simulink model "q1"  (R2020b)
settings: Solver=VariableStepAuto  StartTime=0.0  StopTime=10.0  RelTol=1e-3
settings Model: Creator=MY lenovo  LastModifiedBy=MY lenovo

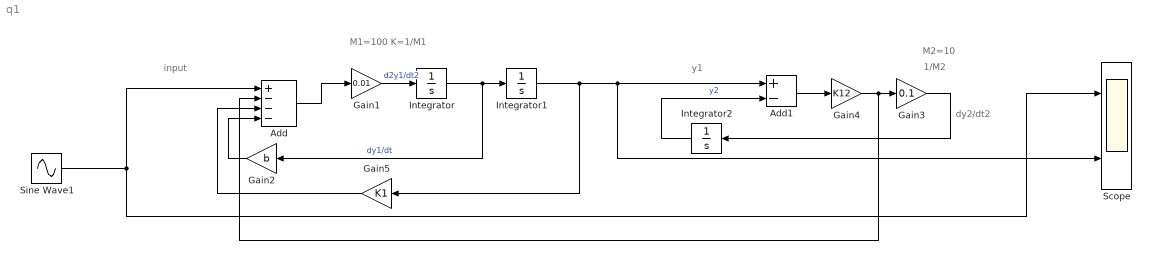
== system q1 ==
  note: M2=10
  note: 1/M2
  note: M1=100
      | K=1/M1
  note: y1
  note: dy2/dt2
  note: input
  Add : Sum  Inputs=+---
  Add1 : Sum  Inputs=+-
  Gain1 : Gain  Gain=0.01
  Gain2 : Gain  Gain=b  mask{b=50}
  Gain3 : Gain  Gain=0.1
  Gain4 : Gain  Gain=K12  mask{K12=1000}
  Gain5 : Gain  Gain=K1  mask{K1=50}
  Integrator : Integrator
  Integrator1 : Integrator
  Integrator2 : Integrator
  Scope : Scope  NumInputPorts=2
  Sine Wave1 : Sin  Amplitude=2  Frequency=10  SampleTime=0
  wires:
  Add1/1 -> Gain4/1
  Gain4/1 -> Gain3/1, Add/2
  Add/1 -> Gain1/1
  Integrator2/1 -> Add1/2  "y2"
  Integrator1/1 -> Gain5/1, Scope/2, Add1/1
  Integrator/1 -> Gain2/1, Integrator1/1  "dy1/dt"
  Gain5/1 -> Add/3
  Gain1/1 -> Integrator/1  "d2y1/dt2"
  Gain2/1 -> Add/4
  Gain3/1 -> Integrator2/1
  Sine Wave1/1 -> Scope/1, Add/1
